simulink library "commdigpbndcpm2"  (Simulink 5.0)
undefined symbols (not defined in the file or in its folder): D
libraries: commblksprivate x14, dspsigattribs x8, commdigbbndcpm2 x8, dspsigops x4, commdigpbndfm2 x2
settings Model: RequirementInfo=9  CovMetricSettings=d  Creator=tdelve  LastModifiedBy=mmclerno

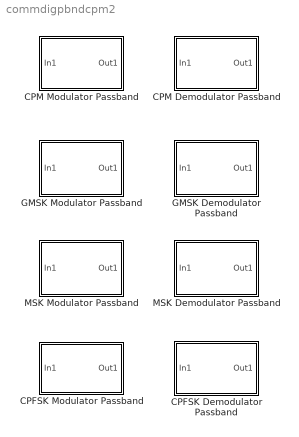
== system commdigpbndcpm2 ==
  CPFSK Demodulator Passband : Subsystem  mask(CPFSK Demodulator Passband){Mnum=4, outputType=Integer, mappingType=Binary, modIdx=.5, td=1/100, numSamp=8, Fc=3000, Ph=0, InSamp=1/8000, traceBack=16}
      mask prompts: Mnum "M-ary number:"; outputType "Output type:"; mappingType "Symbol set ordering:"; modIdx "Modulation index:"; td "Symbol period (s):"; numSamp "Baseband samples per symbol:"; Fc "Carrier frequency (Hz):"; Ph "Carrier initial phase (rad):"; InSamp "Input sample time (s):"; traceBack "Traceback length:"
      mask help:
      | Demodulate the CPFSK modulated input signal using the Viterbi algorithm. Traceback length is the number of trellis branches that the algorithm uses to construct each traceback path.
      |
      | The input must be sample-based.
      |
      | The symbol period divided by the baseband samples per symbol must be an integer multiple of the input sample time.
      mask init:
      | [eStr,params]=commblkpbndcpfskdemod(gcb, 'init');
      | if(eStr.ecode==1)
      |     error(eStr.emsg);
      | elseif(eStr.ecode==2)
      |     warning(eStr.emsg);
      | end;
      settings: RTWFcnNameOpts=Auto  RTWFileNameOpts=Auto
      mask Help: helpview(commbhelp)
      mask StyleString: edit,popup(Bit|Integer),popup(Binary|Gray),edit,edit,edit,edit,edit,edit,edit
      mask CallbackString: |commblkpbndcpfskdemod(gcb,'cbOutputType');||||||||
      mask Display:
      | plot(0,0,100,100,[5+1.5*[[0:.8:10] [10:1.6:20] [20:.8:30]] 50 50 50 50+15*[0 1 1 2 2 3]],[85+10*[sin([0:.8:10]*pi*2/5) sin([10:1.6:20]*pi/5) sin([20:.8:30]*pi*2/5)] 85 99 75 85+8*[1 1 -1 -1 1 1]]);
      | text(50,50,'CPFSK','horiz','center','verti','middle');
  CPFSK Modulator Passband : Subsystem  mask(CPFSK Modulator Passband){Mnum=4, inputType=Integer, mappingType=Binary, modIdx=.5, td=1/100, numSamp=8, Fc=3000, Ph=0, OutSamp=1/8000}
      mask prompts: Mnum "M-ary number:"; inputType "Input type:"; mappingType "Symbol set ordering:"; modIdx "Modulation index:"; td "Symbol period (s):"; numSamp "Baseband samples per symbol:"; Fc "Carrier frequency (Hz):"; Ph "Carrier initial phase (rad):"; OutSamp "Output sample time (s):"
      mask help:
      | Modulate the input signal using continuous phase FSK.
      |
      | The input must be sample-based and contain either an integer or log2(M) bits.
      |
      | The input sample time must equal the symbol period.  Also, the symbol period divided by the baseband samples per symbol must be an integer multiple of the output sample time.
      mask init:
      | [eStr,params]=commblkpbndcpfskmod(gcb, 'init');
      | if(eStr.ecode==1)
      |     error(eStr.emsg);
      | elseif(eStr.ecode==2)
      |     warning(eStr.emsg);
      | end;
      settings: ErrorFcn=commblkpbndcpfskmod  RTWFcnNameOpts=Auto  RTWFileNameOpts=Auto
      mask Help: helpview(commbhelp)
      mask StyleString: edit,popup(Bit|Integer),popup(Binary|Gray),edit,edit,edit,edit,edit,edit
      mask CallbackString: |commblkpbndcpfskmod(gcb,'cbInputType');|||||||
      mask Display:
      | plot(0,0,100,100,[5+15*[0 1 1 2 2 3] 50 50 50 50+1.5*[[0:.8:10] [10:1.6:20] [20:.8:30]]],[85+8*[1 1 -1 -1 1 1] 85 99 75 85+10*[sin([0:.8:10]*pi*2/5) sin([10:1.6:20]*pi/5) sin([20:.8:30]*pi*2/5)]]);
      | text(50,50,'CPFSK','horiz','center','verti','middle');
  CPM Demodulator Passband : Subsystem  mask(CPM Demodulator Passband){Mnum=2, outputType=Integer, mappingType=Binary, modIdx=0.5, pulseShape=Rectangular, BT=0.3, mainLobePulseLength=1, rollOff=0.2, pulseLength=1, preHistory=1, td=1/100, numSamp=8, Fc=3000, Ph=0, InSamp=1/8000, traceBack=16}
      mask prompts: Mnum "M-ary number:"; outputType "Output type:"; mappingType "Symbol set ordering:"; modIdx "Modulation index:"; pulseShape "Frequency pulse shape:"; BT "BT product:"; mainLobePulseLength "Main lobe pulse duration (symbol intervals):"; pulseLength "Pulse length (symbol intervals):"; preHistory "Symbol prehistory:"; td "Symbol period (s):"; numSamp "Baseband samples per symbol:"; Fc "Carrier frequency (Hz):"; Ph "Carrier initial phase (rad):"; InSamp "Input sample time (s):"; traceBack "Traceback length:"
      mask help:
      | Demodulate the CPM modulated input signal using the Viterbi algorithm. Traceback length is the number of trellis branches that the algorithm uses to construct each traceback path.
      |
      | The input must be sample-based.
      |
      | The symbol period divided by the baseband samples per symbol must be an integer multiple of the input sample time.
      mask init:
      | [eStr,params]=commblkpbndcpmdemod(gcb, 'init');
      | if(eStr.ecode==1)
      |     error(eStr.emsg);
      | elseif(eStr.ecode==2)
      |     warning(eStr.emsg);
      | end;
      settings: ErrorFcn=commblkpbndcpmdemod  RTWFcnNameOpts=Auto  RTWFileNameOpts=Auto
      mask Help: helpview(commbhelp)
      mask StyleString: edit,popup(Bit|Integer),popup(Binary|Gray),edit,popup(Rectangular|Raised Cosine|Spectral Raised Cosine|Gaussian|Tamed FM),edit,edit,edit,edit,edit,edit,edit,edit,edit,edit,edit
      mask CallbackString: |commblkpbndcpmdemod(gcb,'cbOutputType');|||commblkpbndcpmdemod(gcb,'cbPulseShape');|||||||||||
      mask Display:
      | plot(0,0,100,100,[5+1.5*[[0:.8:10] [10:1.6:20] [20:.8:30]] 50 50 50 50+15*[0 1 1 2 2 3]],[85+10*[sin([0:.8:10]*pi*2/5) sin([10:1.6:20]*pi/5) sin([20:.8:30]*pi*2/5)] 85 99 75 85+8*[1 1 -1 -1 1 1]]);
      | text(50,50,'CPM','horiz','center','verti','middle');
  CPM Modulator Passband : Subsystem  mask(CPM Modulator Passband){Mnum=2, inputType=Integer, mappingType=Binary, modIdx=0.5, pulseShape=Rectangular, BT=0.3, mainLobePulseLength=1, rollOff=0.2, pulseLength=1, preHistory=1, td=1/100, numSamp=8, Fc=3000, Ph=0, OutSamp=1/8000}
      mask prompts: Mnum "M-ary number:"; inputType "Input type:"; mappingType "Symbol set ordering:"; modIdx "Modulation index:"; pulseShape "Frequency pulse shape:"; BT "BT product:"; mainLobePulseLength "Main lobe pulse duration (symbol intervals):"; pulseLength "Pulse length (symbol intervals):"; preHistory "Symbol prehistory:"; td "Symbol period (s):"; numSamp "Baseband samples per symbol:"; Fc "Carrier frequency (Hz):"; Ph "Carrier initial phase (rad):"; OutSamp "Output sample time (s):"
      mask help:
      | Output the complex envelope representation of the selected continuous phase modulation in response to the input data.
      |
      | The input must be sample-based and contain either an integer or log2(M) bits.
      |
      | The input sample time must equal the symbol period.  Also, the symbol period divided by the baseband samples per symbol must be an integer multiple of the output sample time.
      mask init:
      | [eStr,params]=commblkpbndcpmmod(gcb, 'init');
      | if(eStr.ecode==1)
      |     error(eStr.emsg);
      | elseif(eStr.ecode==2)
      |     warning(eStr.emsg);
      | end;
      settings: ErrorFcn=commblkpbndcpmmod  RTWFcnNameOpts=Auto  RTWFileNameOpts=Auto
      mask Help: helpview(commbhelp)
      mask StyleString: edit,popup(Bit|Integer),popup(Binary|Gray),edit,popup(Rectangular|Raised Cosine|Spectral Raised Cosine|Gaussian|Tamed FM),edit,edit,edit,edit,edit,edit,edit,edit,edit,edit
      mask CallbackString: |commblkpbndcpmmod(gcb,'cbInputType');|||commblkpbndcpmmod(gcb,'cbPulseShape');||||||||||
      mask Display:
      | plot(0,0,100,100,[5+15*[0 1 1 2 2 3] 50 50 50 50+1.5*[[0:.8:10] [10:1.6:20] [20:.8:30]]],[85+8*[1 1 -1 -1 1 1] 85 99 75 85+10*[sin([0:.8:10]*pi*2/5) sin([10:1.6:20]*pi/5) sin([20:.8:30]*pi*2/5)]]);
      | text(50,50,'CPM','horiz','center','verti','middle');
  GMSK Demodulator Passband : Subsystem  mask(GMSK Demodulator Passband){outputType=Integer, BT=.3, pulseLength=4, preHistory=1, td=1/100, numSamp=8, Fc=3000, Ph=0, InSamp=1/8000, traceBack=16}
      mask prompts: outputType "Output type:"; BT "BT product:"; pulseLength "Pulse length (symbol intervals):"; preHistory "Symbol prehistory:"; td "Symbol period (s):"; numSamp "Baseband samples per symbol:"; Fc "Carrier frequency (Hz):"; Ph "Carrier initial phase (rad):"; InSamp "Input sample time (s):"; traceBack "Traceback length:"
      mask help:
      | Demodulate the GMSK modulated input signal using the Viterbi algorithm. Traceback length is the number of trellis branches that the algorithm uses to construct each traceback path.
      |
      | The input must be sample-based.
      |
      | The symbol period divided by the baseband samples per symbol must be an integer multiple of the input sample time.
      mask init:
      | [eStr,params]=commblkpbndgmskdemod(gcb, 'init');
      | if(eStr.ecode==1)
      |     error(eStr.emsg);
      | elseif(eStr.ecode==2)
      |     warning(eStr.emsg);
      | end;
      settings: RTWFcnNameOpts=Auto  RTWFileNameOpts=Auto
      mask Help: helpview(commbhelp)
      mask StyleString: popup(Bit|Integer),edit,edit,edit,edit,edit,edit,edit,edit,edit
      mask Display:
      | plot(0,0,100,100,[5+1.5*[[0:.8:10] [10:1.6:20] [20:.8:30]] 50 50 50 50+15*[0 1 1 2 2 3]],[85+10*[sin([0:.8:10]*pi*2/5) sin([10:1.6:20]*pi/5) sin([20:.8:30]*pi*2/5)] 85 99 75 85+8*[1 1 -1 -1 1 1]]);
      | text(50,50,'GMSK','horiz','center','verti','middle');
  GMSK Modulator Passband : Subsystem  mask(GMSK Modulator Passband){inputType=Integer, BT=.3, pulseLength=4, preHistory=1, td=1/100, numSamp=8, Fc=3000, Ph=0, OutSamp=1/8000}
      mask prompts: inputType "Input type:"; BT "BT product:"; pulseLength "Pulse length (symbol intervals):"; preHistory "Symbol prehistory:"; td "Symbol period (s):"; numSamp "Baseband samples per symbol:"; Fc "Carrier frequency (Hz):"; Ph "Carrier initial phase (rad):"; OutSamp "Output sample time (s):"
      mask help:
      | Modulate the input signal using GMSK.
      |
      | The input must be sample-based and contain either an integer or log2(M) bits.
      |
      | The input sample time must equal the symbol period.  Also, the symbol period divided by the baseband samples per symbol must be an integer multiple of the output sample time.
      mask init:
      | [eStr,params]=commblkpbndgmskmod(gcb, 'init');
      | if(eStr.ecode==1)
      |     error(eStr.emsg);
      | elseif(eStr.ecode==2)
      |     warning(eStr.emsg);
      | end;
      settings: ErrorFcn=commblkpbndgmskmod  RTWFcnNameOpts=Auto  RTWFileNameOpts=Auto
      mask Help: helpview(commbhelp)
      mask StyleString: popup(Bit|Integer),edit,edit,edit,edit,edit,edit,edit,edit
      mask Display:
      | plot(0,0,100,100,[5+15*[0 1 1 2 2 3] 50 50 50 50+1.5*[[0:.8:10] [10:1.6:20] [20:.8:30]]],[85+8*[1 1 -1 -1 1 1] 85 99 75 85+10*[sin([0:.8:10]*pi*2/5) sin([10:1.6:20]*pi/5) sin([20:.8:30]*pi*2/5)]]);
      | text(50,50,'GMSK','horiz','center','verti','middle');
  MSK Demodulator Passband : Subsystem  mask(MSK Demodulator Passband){outputType=Integer, td=1/100, numSamp=8, Fc=3000, Ph=0, InSamp=1/8000, traceBack=16}
      mask prompts: outputType "Output type:"; td "Symbol period (s):"; numSamp "Baseband samples per symbol:"; Fc "Carrier frequency (Hz):"; Ph "Carrier initial phase (rad):"; InSamp "Input sample time (s):"; traceBack "Traceback length:"
      mask help:
      | Demodulate the MSK modulated input signal using the Viterbi algorithm. Traceback length is the number of trellis branches that the algorithm uses to construct each traceback path.
      |
      | The input must be sample-based.
      |
      | The symbol period divided by the baseband samples per symbol must be an integer multiple of the input sample time.
      mask init:
      | [eStr,params]=commblkpbndmskdemod(gcb, 'init');
      | if(eStr.ecode==1)
      |     error(eStr.emsg);
      | elseif(eStr.ecode==2)
      |     warning(eStr.emsg);
      | end;
      settings: RTWFcnNameOpts=Auto  RTWFileNameOpts=Auto
      mask Help: helpview(commbhelp)
      mask StyleString: popup(Bit|Integer),edit,edit,edit,edit,edit,edit
      mask Display:
      | plot(0,0,100,100,[5+1.5*[[0:.8:10] [10:1.6:20] [20:.8:30]] 50 50 50 50+15*[0 1 1 2 2 3]],[85+10*[sin([0:.8:10]*pi*2/5) sin([10:1.6:20]*pi/5) sin([20:.8:30]*pi*2/5)] 85 99 75 85+8*[1 1 -1 -1 1 1]]);
      | text(51,51,'MSK','horiz','center','verti','middle');
  MSK Modulator Passband : Subsystem  mask(MSK Modulator Passband){inputType=Integer, td=1/100, numSamp=8, Fc=3000, Ph=0, OutSamp=1/8000}
      mask prompts: inputType "Input type:"; td "Symbol period (s):"; numSamp "Baseband samples per symbol:"; Fc "Carrier frequency (Hz):"; Ph "Carrier initial phase (rad):"; OutSamp "Output sample time (s):"
      mask help:
      | Modulate the input signal using MSK.
      |
      | The input must be sample-based and contain either an integer or log2(M) bits.
      |
      | The input sample time must equal the symbol period.  Also, the symbol period divided by the baseband samples per symbol must be an integer multiple of the output sample time.
      mask init:
      | [eStr,params]=commblkpbndmskmod(gcb, 'init');
      | if(eStr.ecode==1)
      |     error(eStr.emsg);
      | elseif(eStr.ecode==2)
      |     warning(eStr.emsg);
      | end;
      settings: ErrorFcn=commblkpbndmskmod  RTWFcnNameOpts=Auto  RTWFileNameOpts=Auto
      mask Help: helpview(commbhelp)
      mask StyleString: popup(Bit|Integer),edit,edit,edit,edit,edit
      mask Display:
      | plot(0,0,100,100,[5+15*[0 1 1 2 2 3] 50 50 50 50+1.5*[[0:.8:10] [10:1.6:20] [20:.8:30]]],[85+8*[1 1 -1 -1 1 1] 85 99 75 85+10*[sin([0:.8:10]*pi*2/5) sin([10:1.6:20]*pi/5) sin([20:.8:30]*pi*2/5)]]);
      | text(51,51,'MSK','horiz','center','verti','middle');

== system commdigpbndcpm2/CPFSK Demodulator Passband ==
  In1 : Inport  Port=1  LatchInput=off
  CPM Demodulator Passband : Subsystem  AncestorBlock=|  mask(CPM Demodulator Passband){Mnum=Mnum, outputType=Integer, mappingType=Binary, modIdx=modIdx, pulseShape=Rectangular, BT=0.3, mainLobePulseLength=1, rollOff=0.2, pulseLength=1, preHistory=1, td=td, numSamp=numSamp, Fc=Fc, Ph=Ph, InSamp=InSamp, traceBack=traceBack}
      | commdigpbndcpm2/CPM
      | Demodulator
      | Passband
      mask prompts: Mnum "M-ary number:"; outputType "Output type:"; mappingType "Symbol set ordering:"; modIdx "Modulation index:"; pulseShape "Frequency pulse shape:"; BT "BT product:"; mainLobePulseLength "Main lobe pulse duration (symbol intervals):"; pulseLength "Pulse length (symbol intervals):"; preHistory "Symbol prehistory:"; td "Symbol period (s):"; numSamp "Baseband samples per symbol:"; Fc "Carrier frequency (Hz):"; Ph "Carrier initial phase (rad):"; InSamp "Input sample time (s):"; traceBack "Traceback length:"
      mask help:
      | Demodulate the CPM modulated input signal using the Viterbi algorithm. Traceback length is the number of trellis branches that the algorithm uses to construct each traceback path.
      |
      | The input must be sample-based.
      mask init:
      | [eStr,params]=commblkpbndcpmdemod(gcb, 'init');
      | if(eStr.ecode==1)
      |     error(eStr.emsg);
      | elseif(eStr.ecode==2)
      |     warning(eStr.emsg);
      | end;
      settings: ErrorFcn=commblkpbndcpmdemod  RTWFcnNameOpts=Auto  RTWFileNameOpts=Auto
      mask Help: helpview(commbhelp)
      mask StyleString: edit,popup(Bit|Integer),popup(Binary|Gray),edit,popup(Rectangular|Raised Cosine|Spectral Raised Cosine|Gaussian|Tamed FM),edit,edit,edit,edit,edit,edit,edit,edit,edit,edit,edit
      mask CallbackString: |commblkpbndcpmdemod(gcb,'cbOutputType');|||commblkpbndcpmdemod(gcb,'cbPulseShape');|||||||||||
      mask Display:
      | plot(0,0,100,100,[5+1.5*[[0:.8:10] [10:1.6:20] [20:.8:30]] 50 50 50 50+15*[0 1 1 2 2 3]],[85+10*[sin([0:.8:10]*pi*2/5) sin([10:1.6:20]*pi/5) sin([20:.8:30]*pi*2/5)] 85 99 75 85+8*[1 1 -1 -1 1 1]]);
      | text(50,50,'CPM','horiz','center','verti','middle');
  Out1 : Outport  Port=1
  wires:
  CPM Demodulator Passband/1(Out1) -> Out1/1
  In1/1 -> CPM Demodulator Passband/1(In1)

== system commdigpbndcpm2/CPFSK Modulator Passband ==
  In1 : Inport  Port=1  LatchInput=off
  CPM Modulator Passband : Subsystem  AncestorBlock=|  mask(CPM Modulator Passband){Mnum=Mnum, inputType=Integer, mappingType=Binary, modIdx=modIdx, pulseShape=Rectangular, BT=0.3, mainLobePulseLength=1, rollOff=0.2, pulseLength=1, preHistory=1, td=td, numSamp=numSamp, Fc=Fc, Ph=Ph, OutSamp=OutSamp}
      | commdigpbndcpm2/CPM
      | Modulator
      | Passband
      mask prompts: Mnum "M-ary number:"; inputType "Input type:"; mappingType "Symbol set ordering:"; modIdx "Modulation index:"; pulseShape "Frequency pulse shape:"; BT "BT product:"; mainLobePulseLength "Main lobe pulse duration (symbol intervals):"; pulseLength "Pulse length (symbol intervals):"; preHistory "Symbol prehistory:"; td "Symbol period (s):"; numSamp "Baseband samples per symbol:"; Fc "Carrier frequency (Hz):"; Ph "Carrier initial phase (rad):"; OutSamp "Output sample time:"
      mask help:
      | Output the complex envelope representation of the selected continuous phase modulation in response to the input data.
      |
      | The input must be sample-based and contain either an integer or log2(M) bits. The input sample time must equal the symbol period.
      mask init:
      | [eStr,params]=commblkpbndcpmmod(gcb, 'init');
      | if(eStr.ecode==1)
      |     error(eStr.emsg);
      | elseif(eStr.ecode==2)
      |     warning(eStr.emsg);
      | end;
      settings: ErrorFcn=commblkpbndcpmmod  RTWFcnNameOpts=Auto  RTWFileNameOpts=Auto
      mask Help: helpview(commbhelp)
      mask StyleString: edit,popup(Bit|Integer),popup(Binary|Gray),edit,popup(Rectangular|Raised Cosine|Spectral Raised Cosine|Gaussian|Tamed FM),edit,edit,edit,edit,edit,edit,edit,edit,edit,edit
      mask CallbackString: |commblkpbndcpmmod(gcb,'cbInputType');|||commblkpbndcpmmod(gcb,'cbPulseShape');||||||||||
      mask Display:
      | plot(0,0,100,100,[5+15*[0 1 1 2 2 3] 50 50 50 50+1.5*[[0:.8:10] [10:1.6:20] [20:.8:30]]],[85+8*[1 1 -1 -1 1 1] 85 99 75 85+10*[sin([0:.8:10]*pi*2/5) sin([10:1.6:20]*pi/5) sin([20:.8:30]*pi*2/5)]]);
      | text(50,50,'CPM','horiz','center','verti','middle');
  Out1 : Outport  Port=1
  wires:
  CPM Modulator Passband/1(Out1) -> Out1/1
  In1/1 -> CPM Modulator Passband/1(In1)

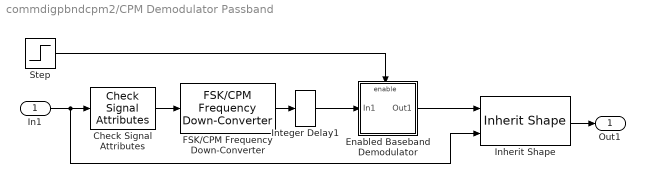
== system commdigpbndcpm2/CPM Demodulator Passband ==
  In1 : Inport  Port=1  LatchInput=off
  Check Signal Attributes : dspsigattribs/Check Signal Attributes  SigAttribCheckMethod=Matches attributes exactly  Complexity=Ignore  Frame=Frame-based  DimsCheckMethod=Ignore  Dimensions=1-D  DatatypeCheckMethod=Ignore  DatatypeGeneral=Boolean  DtypeFloatSpecific=Any floating-point  DtypeFixedSpecific=Any fixed-point  DtypeIntSpecific=Any integer  SampleMode=Ignore
  Enabled Baseband Demodulator : Subsystem  TreatAsAtomicUnit=on
      settings: RTWFcnNameOpts=Auto  RTWFileNameOpts=Auto
  FSK/CPM Frequency Down-Converter : commblksprivate/FSK//CPM Frequency Down-Converter  modType=CPM  M=8  freqSep=100  td=td  Fc=Fc  Ph=Ph  Tin=InSamp  Tout=td / numSamp
  Inherit Shape : commblksprivate/Inherit Shape
  Integer Delay1 : dspsigops/Integer Delay  delay=numSamp-1  ic=0
  Step : Step  Time=td  Before=0  After=1  SampleTime=td
  Out1 : Outport  Port=1
  wires:
  Check Signal Attributes/1 -> FSK/CPM Frequency Down-Converter/1
  FSK/CPM Frequency Down-Converter/1 -> Integer Delay1/1
  Enabled Baseband Demodulator/1(Out1) -> Inherit Shape/1
  In1/1 -> Check Signal Attributes/1, Inherit Shape/2
  Inherit Shape/1 -> Out1/1
  Integer Delay1/1 -> Enabled Baseband Demodulator/1(In1)
  Step/1 -> Enabled Baseband Demodulator/Enable

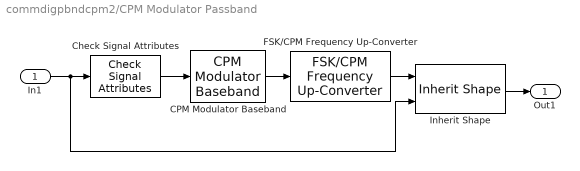
== system commdigpbndcpm2/CPM Modulator Passband ==
  In1 : Inport  Port=1  LatchInput=off
  CPM Modulator Baseband : commdigbbndcpm2/CPM Modulator Baseband  Mnum=Mnum  inputType=Integer  mappingType=Binary  modIdx=modIdx  pulseShape=Rectangular  BT=BT  mainLobePulseLength=1  rollOff=rollOff  pulseLength=pulseLength  preHistory=preHistory  phaseOffset=0  samplesPerSymbol=numSamp
  Check Signal Attributes : dspsigattribs/Check Signal Attributes  SigAttribCheckMethod=Matches attributes exactly  Complexity=Ignore  Frame=Frame-based  DimsCheckMethod=Ignore  Dimensions=1-D  DatatypeCheckMethod=Ignore  DatatypeGeneral=Boolean  DtypeFloatSpecific=Any floating-point  DtypeFixedSpecific=Any fixed-point  DtypeIntSpecific=Any integer  SampleMode=Ignore
  FSK/CPM Frequency Up-Converter : commblksprivate/FSK//CPM Frequency Up-Converter  modType=CPM  M=8  freqSep=6  td=td  Fc=Fc  Ph=Ph  Tin=td / numSamp  Tout=OutSamp
  Inherit Shape : commblksprivate/Inherit Shape
  Out1 : Outport  Port=1
  wires:
  FSK/CPM Frequency Up-Converter/1 -> Inherit Shape/1
  CPM Modulator Baseband/1 -> FSK/CPM Frequency Up-Converter/1
  Check Signal Attributes/1 -> CPM Modulator Baseband/1
  In1/1 -> Check Signal Attributes/1, Inherit Shape/2
  Inherit Shape/1 -> Out1/1

== system commdigpbndcpm2/GMSK Demodulator Passband ==
  In1 : Inport  Port=1  LatchInput=off
  CPM Demodulator Passband : Subsystem  AncestorBlock=|  mask(CPM Demodulator Passband){Mnum=2, outputType=Integer, mappingType=Binary, modIdx=0.5, pulseShape=Gaussian, BT=BT, mainLobePulseLength=1, rollOff=0.2, pulseLength=pulseLength, preHistory=preHistory, td=td, numSamp=numSamp, Fc=Fc, Ph=Ph, InSamp=InSamp, traceBack=traceBack}
      | commdigpbndcpm2/CPM
      | Demodulator
      | Passband
      mask prompts: Mnum "M-ary number:"; outputType "Output type:"; mappingType "Symbol set ordering:"; modIdx "Modulation index:"; pulseShape "Frequency pulse shape:"; BT "BT product:"; mainLobePulseLength "Main lobe pulse duration (symbol intervals):"; pulseLength "Pulse length (symbol intervals):"; preHistory "Symbol prehistory:"; td "Symbol period (s):"; numSamp "Baseband samples per symbol:"; Fc "Carrier frequency (Hz):"; Ph "Carrier initial phase (rad):"; InSamp "Input sample time (s):"; traceBack "Traceback length:"
      mask help:
      | Demodulate the CPM modulated input signal using the Viterbi algorithm. Traceback length is the number of trellis branches that the algorithm uses to construct each traceback path.
      |
      | The input must be sample-based.
      mask init:
      | [eStr,params]=commblkpbndcpmdemod(gcb, 'init');
      | if(eStr.ecode==1)
      |     error(eStr.emsg);
      | elseif(eStr.ecode==2)
      |     warning(eStr.emsg);
      | end;
      settings: ErrorFcn=commblkpbndcpmdemod  RTWFcnNameOpts=Auto  RTWFileNameOpts=Auto
      mask Help: helpview(commbhelp)
      mask StyleString: edit,popup(Bit|Integer),popup(Binary|Gray),edit,popup(Rectangular|Raised Cosine|Spectral Raised Cosine|Gaussian|Tamed FM),edit,edit,edit,edit,edit,edit,edit,edit,edit,edit,edit
      mask CallbackString: |commblkpbndcpmdemod(gcb,'cbOutputType');|||commblkpbndcpmdemod(gcb,'cbPulseShape');|||||||||||
      mask Display:
      | plot(0,0,100,100,[5+1.5*[[0:.8:10] [10:1.6:20] [20:.8:30]] 50 50 50 50+15*[0 1 1 2 2 3]],[85+10*[sin([0:.8:10]*pi*2/5) sin([10:1.6:20]*pi/5) sin([20:.8:30]*pi*2/5)] 85 99 75 85+8*[1 1 -1 -1 1 1]]);
      | text(50,50,'CPM','horiz','center','verti','middle');
  Out1 : Outport  Port=1
  wires:
  CPM Demodulator Passband/1(Out1) -> Out1/1
  In1/1 -> CPM Demodulator Passband/1(In1)

== system commdigpbndcpm2/GMSK Modulator Passband ==
  In1 : Inport  Port=1  LatchInput=off
  CPM Modulator Passband : Subsystem  AncestorBlock=|  mask(CPM Modulator Passband){Mnum=2, inputType=Integer, mappingType=Binary, modIdx=.5, pulseShape=Gaussian, BT=BT, mainLobePulseLength=1, rollOff=0.2, pulseLength=pulseLength, preHistory=preHistory, td=td, numSamp=numSamp, Fc=Fc, Ph=Ph, OutSamp=OutSamp}
      | commdigpbndcpm2/CPM
      | Modulator
      | Passband
      mask prompts: Mnum "M-ary number:"; inputType "Input type:"; mappingType "Symbol set ordering:"; modIdx "Modulation index:"; pulseShape "Frequency pulse shape:"; BT "BT product:"; mainLobePulseLength "Main lobe pulse duration (symbol intervals):"; pulseLength "Pulse length (symbol intervals):"; preHistory "Symbol prehistory:"; td "Symbol period (s):"; numSamp "Baseband samples per symbol:"; Fc "Carrier frequency (Hz):"; Ph "Carrier initial phase (rad):"; OutSamp "Output sample time:"
      mask help:
      | Output the complex envelope representation of the selected continuous phase modulation in response to the input data.
      |
      | The input must be sample-based and contain either an integer or log2(M) bits. The input sample time must equal the symbol period.
      mask init:
      | [eStr,params]=commblkpbndcpmmod(gcb, 'init');
      | if(eStr.ecode==1)
      |     error(eStr.emsg);
      | elseif(eStr.ecode==2)
      |     warning(eStr.emsg);
      | end;
      settings: ErrorFcn=commblkpbndcpmmod  RTWFcnNameOpts=Auto  RTWFileNameOpts=Auto
      mask Help: helpview(commbhelp)
      mask StyleString: edit,popup(Bit|Integer),popup(Binary|Gray),edit,popup(Rectangular|Raised Cosine|Spectral Raised Cosine|Gaussian|Tamed FM),edit,edit,edit,edit,edit,edit,edit,edit,edit,edit
      mask CallbackString: |commblkpbndcpmmod(gcb,'cbInputType');|||commblkpbndcpmmod(gcb,'cbPulseShape');||||||||||
      mask Display:
      | plot(0,0,100,100,[5+15*[0 1 1 2 2 3] 50 50 50 50+1.5*[[0:.8:10] [10:1.6:20] [20:.8:30]]],[85+8*[1 1 -1 -1 1 1] 85 99 75 85+10*[sin([0:.8:10]*pi*2/5) sin([10:1.6:20]*pi/5) sin([20:.8:30]*pi*2/5)]]);
      | text(50,50,'CPM','horiz','center','verti','middle');
  Out1 : Outport  Port=1
  wires:
  CPM Modulator Passband/1(Out1) -> Out1/1
  In1/1 -> CPM Modulator Passband/1(In1)

== system commdigpbndcpm2/MSK Demodulator Passband ==
  In1 : Inport  Port=1  LatchInput=off
  CPM Demodulator Passband : Subsystem  AncestorBlock=|  mask(CPM Demodulator Passband){Mnum=2, outputType=Integer, mappingType=Binary, modIdx=0.5, pulseShape=Rectangular, BT=0.3, mainLobePulseLength=1, rollOff=0.2, pulseLength=1, preHistory=1, td=td, numSamp=numSamp, Fc=Fc, Ph=Ph, InSamp=InSamp, traceBack=traceBack}
      | commdigpbndcpm2/CPM
      | Demodulator
      | Passband
      mask prompts: Mnum "M-ary number:"; outputType "Output type:"; mappingType "Symbol set ordering:"; modIdx "Modulation index:"; pulseShape "Frequency pulse shape:"; BT "BT product:"; mainLobePulseLength "Main lobe pulse duration (symbol intervals):"; pulseLength "Pulse length (symbol intervals):"; preHistory "Symbol prehistory:"; td "Symbol period (s):"; numSamp "Baseband samples per symbol:"; Fc "Carrier frequency (Hz):"; Ph "Carrier initial phase (rad):"; InSamp "Input sample time (s):"; traceBack "Traceback length:"
      mask help:
      | Demodulate the CPM modulated input signal using the Viterbi algorithm. Traceback length is the number of trellis branches that the algorithm uses to construct each traceback path.
      |
      | The input must be sample-based.
      mask init:
      | [eStr,params]=commblkpbndcpmdemod(gcb, 'init');
      | if(eStr.ecode==1)
      |     error(eStr.emsg);
      | elseif(eStr.ecode==2)
      |     warning(eStr.emsg);
      | end;
      settings: ErrorFcn=commblkpbndcpmdemod  RTWFcnNameOpts=Auto  RTWFileNameOpts=Auto
      mask Help: helpview(commbhelp)
      mask StyleString: edit,popup(Bit|Integer),popup(Binary|Gray),edit,popup(Rectangular|Raised Cosine|Spectral Raised Cosine|Gaussian|Tamed FM),edit,edit,edit,edit,edit,edit,edit,edit,edit,edit,edit
      mask CallbackString: |commblkpbndcpmdemod(gcb,'cbOutputType');|||commblkpbndcpmdemod(gcb,'cbPulseShape');|||||||||||
      mask Display:
      | plot(0,0,100,100,[5+1.5*[[0:.8:10] [10:1.6:20] [20:.8:30]] 50 50 50 50+15*[0 1 1 2 2 3]],[85+10*[sin([0:.8:10]*pi*2/5) sin([10:1.6:20]*pi/5) sin([20:.8:30]*pi*2/5)] 85 99 75 85+8*[1 1 -1 -1 1 1]]);
      | text(50,50,'CPM','horiz','center','verti','middle');
  Out1 : Outport  Port=1
  wires:
  CPM Demodulator Passband/1(Out1) -> Out1/1
  In1/1 -> CPM Demodulator Passband/1(In1)

== system commdigpbndcpm2/MSK Modulator Passband ==
  In1 : Inport  Port=1  LatchInput=off
  CPM Modulator Passband : Subsystem  AncestorBlock=|  mask(CPM Modulator Passband){Mnum=2, inputType=Integer, mappingType=Binary, modIdx=0.5, pulseShape=Rectangular, BT=0.3, mainLobePulseLength=1, rollOff=0.2, pulseLength=1, preHistory=1, td=td, numSamp=numSamp, Fc=Fc, Ph=Ph, OutSamp=OutSamp}
      | commdigpbndcpm2/CPM
      | Modulator
      | Passband
      mask prompts: Mnum "M-ary number:"; inputType "Input type:"; mappingType "Symbol set ordering:"; modIdx "Modulation index:"; pulseShape "Frequency pulse shape:"; BT "BT product:"; mainLobePulseLength "Main lobe pulse duration (symbol intervals):"; pulseLength "Pulse length (symbol intervals):"; preHistory "Symbol prehistory:"; td "Symbol period (s):"; numSamp "Baseband samples per symbol:"; Fc "Carrier frequency (Hz):"; Ph "Carrier initial phase (rad):"; OutSamp "Output sample time:"
      mask help:
      | Output the complex envelope representation of the selected continuous phase modulation in response to the input data.
      |
      | The input must be sample-based and contain either an integer or log2(M) bits. The input sample time must equal the symbol period.
      mask init:
      | [eStr,params]=commblkpbndcpmmod(gcb, 'init');
      | if(eStr.ecode==1)
      |     error(eStr.emsg);
      | elseif(eStr.ecode==2)
      |     warning(eStr.emsg);
      | end;
      settings: ErrorFcn=commblkpbndcpmmod  RTWFcnNameOpts=Auto  RTWFileNameOpts=Auto
      mask Help: helpview(commbhelp)
      mask StyleString: edit,popup(Bit|Integer),popup(Binary|Gray),edit,popup(Rectangular|Raised Cosine|Spectral Raised Cosine|Gaussian|Tamed FM),edit,edit,edit,edit,edit,edit,edit,edit,edit,edit
      mask CallbackString: |commblkpbndcpmmod(gcb,'cbInputType');|||commblkpbndcpmmod(gcb,'cbPulseShape');||||||||||
      mask Display:
      | plot(0,0,100,100,[5+15*[0 1 1 2 2 3] 50 50 50 50+1.5*[[0:.8:10] [10:1.6:20] [20:.8:30]]],[85+8*[1 1 -1 -1 1 1] 85 99 75 85+10*[sin([0:.8:10]*pi*2/5) sin([10:1.6:20]*pi/5) sin([20:.8:30]*pi*2/5)]]);
      | text(50,50,'CPM','horiz','center','verti','middle');
  Out1 : Outport  Port=1
  wires:
  CPM Modulator Passband/1(Out1) -> Out1/1
  In1/1 -> CPM Modulator Passband/1(In1)

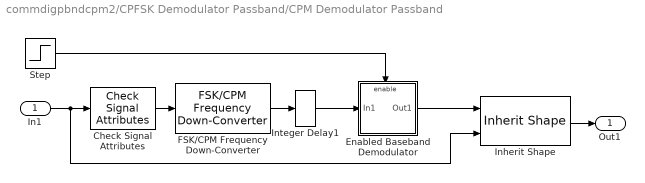
== system commdigpbndcpm2/CPFSK Demodulator Passband/CPM Demodulator Passband ==
  In1 : Inport  Port=1  LatchInput=off
  Check Signal Attributes : dspsigattribs/Check Signal Attributes  SigAttribCheckMethod=Matches attributes exactly  Complexity=Ignore  Frame=Frame-based  DimsCheckMethod=Ignore  Dimensions=1-D  DatatypeCheckMethod=Ignore  DatatypeGeneral=Boolean  DtypeFloatSpecific=Any floating-point  DtypeFixedSpecific=Any fixed-point  DtypeIntSpecific=Any integer  SampleMode=Ignore
  Enabled Baseband Demodulator : Subsystem  TreatAsAtomicUnit=on
      settings: RTWFcnNameOpts=Auto  RTWFileNameOpts=Auto
  FSK/CPM Frequency Down-Converter : commblksprivate/FSK//CPM Frequency Down-Converter  AncestorBlock=|  modType=CPM  M=8  freqSep=100  td=td  Fc=Fc  Ph=Ph  Tin=InSamp  Tout=td / numSamp
      | commblksprivate/PAM//QAM//PSK
      | Frequency
      | Down-Converter
  Inherit Shape : commblksprivate/Inherit Shape
  Integer Delay1 : dspsigops/Integer Delay  delay=numSamp-1  ic=0
  Step : Step  Time=td  Before=0  After=1  SampleTime=td
  Out1 : Outport  Port=1
  wires:
  Step/1 -> Enabled Baseband Demodulator/Enable
  Integer Delay1/1 -> Enabled Baseband Demodulator/1(In1)
  Inherit Shape/1 -> Out1/1
  In1/1 -> Inherit Shape/2, Check Signal Attributes/1
  Enabled Baseband Demodulator/1(Out1) -> Inherit Shape/1
  FSK/CPM Frequency Down-Converter/1 -> Integer Delay1/1
  Check Signal Attributes/1 -> FSK/CPM Frequency Down-Converter/1

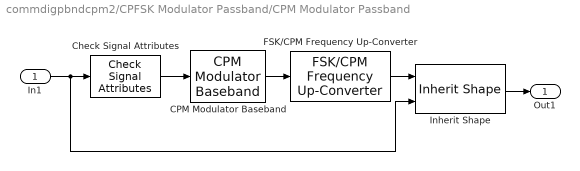
== system commdigpbndcpm2/CPFSK Modulator Passband/CPM Modulator Passband ==
  In1 : Inport  Port=1  LatchInput=off
  CPM Modulator Baseband : commdigbbndcpm2/CPM Modulator Baseband  Mnum=Mnum  inputType=Integer  mappingType=Binary  modIdx=modIdx  pulseShape=Rectangular  BT=BT  mainLobePulseLength=1  rollOff=rollOff  pulseLength=pulseLength  preHistory=preHistory  phaseOffset=0  samplesPerSymbol=numSamp
  Check Signal Attributes : dspsigattribs/Check Signal Attributes  SigAttribCheckMethod=Matches attributes exactly  Complexity=Ignore  Frame=Frame-based  DimsCheckMethod=Ignore  Dimensions=1-D  DatatypeCheckMethod=Ignore  DatatypeGeneral=Boolean  DtypeFloatSpecific=Any floating-point  DtypeFixedSpecific=Any fixed-point  DtypeIntSpecific=Any integer  SampleMode=Ignore
  FSK/CPM Frequency Up-Converter : commdigpbndfm2/M-FSK Modulator Passband/FSK//CPM Frequency Up-Converter  AncestorBlock=|  modType=CPM  M=8  freqSep=6  td=td  Fc=Fc  Ph=Ph  Tin=td / numSamp  Tout=OutSamp
      | commblksprivate/FSK//CPM
      | Frequency
      | Up-Converter
  Inherit Shape : commblksprivate/Inherit Shape
  Out1 : Outport  Port=1
  wires:
  Inherit Shape/1 -> Out1/1
  In1/1 -> Inherit Shape/2, Check Signal Attributes/1
  Check Signal Attributes/1 -> CPM Modulator Baseband/1
  CPM Modulator Baseband/1 -> FSK/CPM Frequency Up-Converter/1
  FSK/CPM Frequency Up-Converter/1 -> Inherit Shape/1

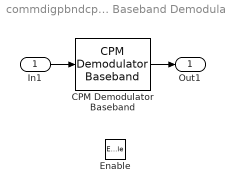
== system commdigpbndcpm2/CPM Demodulator Passband/Enabled Baseband Demodulator ==
  In1 : Inport  Port=1  LatchInput=off
  Enable : EnablePort
  CPM Demodulator Baseband : commdigbbndcpm2/CPM Demodulator Baseband  Mnum=Mnum  outputType=Integer  mappingType=Binary  modIdx=modIdx  pulseShape=Rectangular  BT=BT  mainLobePulseLength=1  rollOff=rollOff  pulseLength=pulseLength  preHistory=preHistory  phaseOffset=0  samplesPerSymbol=numSamp  traceBack=traceBack
  Out1 : Outport  Port=1
  wires:
  CPM Demodulator Baseband/1 -> Out1/1
  In1/1 -> CPM Demodulator Baseband/1

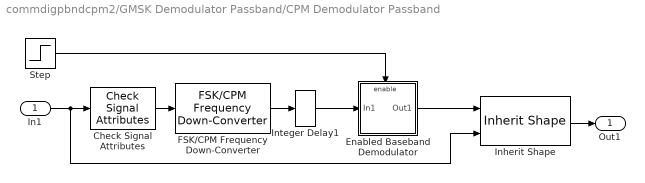
== system commdigpbndcpm2/GMSK Demodulator Passband/CPM Demodulator Passband ==
  In1 : Inport  Port=1  LatchInput=off
  Check Signal Attributes : dspsigattribs/Check Signal Attributes  SigAttribCheckMethod=Matches attributes exactly  Complexity=Ignore  Frame=Frame-based  DimsCheckMethod=Ignore  Dimensions=1-D  DatatypeCheckMethod=Ignore  DatatypeGeneral=Boolean  DtypeFloatSpecific=Any floating-point  DtypeFixedSpecific=Any fixed-point  DtypeIntSpecific=Any integer  SampleMode=Ignore
  Enabled Baseband Demodulator : Subsystem  TreatAsAtomicUnit=on
      settings: RTWFcnNameOpts=Auto  RTWFileNameOpts=Auto
  FSK/CPM Frequency Down-Converter : commblksprivate/FSK//CPM Frequency Down-Converter  AncestorBlock=|  modType=CPM  M=8  freqSep=100  td=td  Fc=Fc  Ph=Ph  Tin=InSamp  Tout=td / numSamp
      | commblksprivate/PAM//QAM//PSK
      | Frequency
      | Down-Converter
  Inherit Shape : commblksprivate/Inherit Shape
  Integer Delay1 : dspsigops/Integer Delay  delay=numSamp-1  ic=0
  Step : Step  Time=td  Before=0  After=1  SampleTime=td
  Out1 : Outport  Port=1
  wires:
  Step/1 -> Enabled Baseband Demodulator/Enable
  Integer Delay1/1 -> Enabled Baseband Demodulator/1(In1)
  Inherit Shape/1 -> Out1/1
  In1/1 -> Inherit Shape/2, Check Signal Attributes/1
  Enabled Baseband Demodulator/1(Out1) -> Inherit Shape/1
  FSK/CPM Frequency Down-Converter/1 -> Integer Delay1/1
  Check Signal Attributes/1 -> FSK/CPM Frequency Down-Converter/1

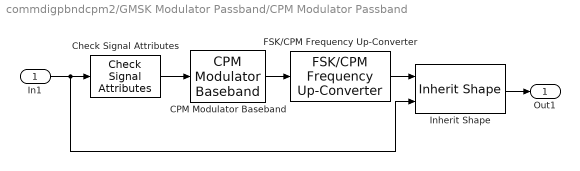
== system commdigpbndcpm2/GMSK Modulator Passband/CPM Modulator Passband ==
  In1 : Inport  Port=1  LatchInput=off
  CPM Modulator Baseband : commdigbbndcpm2/CPM Modulator Baseband  Mnum=Mnum  inputType=Integer  mappingType=Binary  modIdx=modIdx  pulseShape=Gaussian  BT=BT  mainLobePulseLength=1  rollOff=rollOff  pulseLength=pulseLength  preHistory=preHistory  phaseOffset=0  samplesPerSymbol=numSamp
  Check Signal Attributes : dspsigattribs/Check Signal Attributes  SigAttribCheckMethod=Matches attributes exactly  Complexity=Ignore  Frame=Frame-based  DimsCheckMethod=Ignore  Dimensions=1-D  DatatypeCheckMethod=Ignore  DatatypeGeneral=Boolean  DtypeFloatSpecific=Any floating-point  DtypeFixedSpecific=Any fixed-point  DtypeIntSpecific=Any integer  SampleMode=Ignore
  FSK/CPM Frequency Up-Converter : commdigpbndfm2/M-FSK Modulator Passband/FSK//CPM Frequency Up-Converter  AncestorBlock=|  modType=CPM  M=8  freqSep=6  td=td  Fc=Fc  Ph=Ph  Tin=td / numSamp  Tout=OutSamp
      | commblksprivate/FSK//CPM
      | Frequency
      | Up-Converter
  Inherit Shape : commblksprivate/Inherit Shape
  Out1 : Outport  Port=1
  wires:
  Inherit Shape/1 -> Out1/1
  In1/1 -> Inherit Shape/2, Check Signal Attributes/1
  Check Signal Attributes/1 -> CPM Modulator Baseband/1
  CPM Modulator Baseband/1 -> FSK/CPM Frequency Up-Converter/1
  FSK/CPM Frequency Up-Converter/1 -> Inherit Shape/1

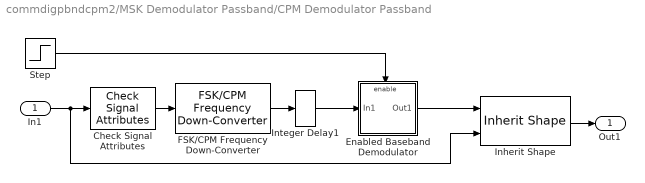
== system commdigpbndcpm2/MSK Demodulator Passband/CPM Demodulator Passband ==
  In1 : Inport  Port=1  LatchInput=off
  Check Signal Attributes : dspsigattribs/Check Signal Attributes  SigAttribCheckMethod=Matches attributes exactly  Complexity=Ignore  Frame=Frame-based  DimsCheckMethod=Ignore  Dimensions=1-D  DatatypeCheckMethod=Ignore  DatatypeGeneral=Boolean  DtypeFloatSpecific=Any floating-point  DtypeFixedSpecific=Any fixed-point  DtypeIntSpecific=Any integer  SampleMode=Ignore
  Enabled Baseband Demodulator : Subsystem  TreatAsAtomicUnit=on
      settings: RTWFcnNameOpts=Auto  RTWFileNameOpts=Auto
  FSK/CPM Frequency Down-Converter : commblksprivate/FSK//CPM Frequency Down-Converter  AncestorBlock=|  modType=CPM  M=8  freqSep=100  td=td  Fc=Fc  Ph=Ph  Tin=InSamp  Tout=td / numSamp
      | commblksprivate/PAM//QAM//PSK
      | Frequency
      | Down-Converter
  Inherit Shape : commblksprivate/Inherit Shape
  Integer Delay1 : dspsigops/Integer Delay  delay=numSamp-1  ic=0
  Step : Step  Time=td  Before=0  After=1  SampleTime=td
  Out1 : Outport  Port=1
  wires:
  Step/1 -> Enabled Baseband Demodulator/Enable
  Integer Delay1/1 -> Enabled Baseband Demodulator/1(In1)
  Inherit Shape/1 -> Out1/1
  In1/1 -> Inherit Shape/2, Check Signal Attributes/1
  Enabled Baseband Demodulator/1(Out1) -> Inherit Shape/1
  FSK/CPM Frequency Down-Converter/1 -> Integer Delay1/1
  Check Signal Attributes/1 -> FSK/CPM Frequency Down-Converter/1

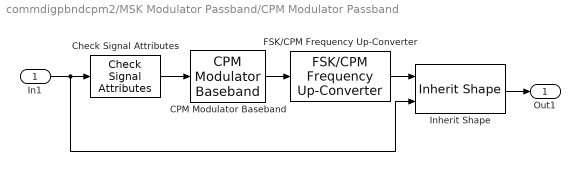
== system commdigpbndcpm2/MSK Modulator Passband/CPM Modulator Passband ==
  In1 : Inport  Port=1  LatchInput=off
  CPM Modulator Baseband : commdigbbndcpm2/CPM Modulator Baseband  Mnum=Mnum  inputType=Integer  mappingType=Binary  modIdx=modIdx  pulseShape=Rectangular  BT=BT  mainLobePulseLength=1  rollOff=rollOff  pulseLength=pulseLength  preHistory=preHistory  phaseOffset=0  samplesPerSymbol=numSamp
  Check Signal Attributes : dspsigattribs/Check Signal Attributes  SigAttribCheckMethod=Matches attributes exactly  Complexity=Ignore  Frame=Frame-based  DimsCheckMethod=Ignore  Dimensions=1-D  DatatypeCheckMethod=Ignore  DatatypeGeneral=Boolean  DtypeFloatSpecific=Any floating-point  DtypeFixedSpecific=Any fixed-point  DtypeIntSpecific=Any integer  SampleMode=Ignore
  FSK/CPM Frequency Up-Converter : commblksprivate/FSK//CPM Frequency Up-Converter  modType=CPM  M=8  freqSep=6  td=td  Fc=Fc  Ph=Ph  Tin=td / numSamp  Tout=OutSamp
  Inherit Shape : commblksprivate/Inherit Shape
  Out1 : Outport  Port=1
  wires:
  Inherit Shape/1 -> Out1/1
  In1/1 -> Inherit Shape/2, Check Signal Attributes/1
  Check Signal Attributes/1 -> CPM Modulator Baseband/1
  CPM Modulator Baseband/1 -> FSK/CPM Frequency Up-Converter/1
  FSK/CPM Frequency Up-Converter/1 -> Inherit Shape/1

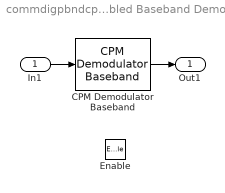
== system commdigpbndcpm2/CPFSK Demodulator Passband/CPM Demodulator Passband/Enabled Baseband Demodulator ==
  In1 : Inport  Port=1  LatchInput=off
  Enable : EnablePort
  CPM Demodulator Baseband : commdigbbndcpm2/CPM Demodulator Baseband  Mnum=Mnum  outputType=Integer  mappingType=Binary  modIdx=modIdx  pulseShape=Rectangular  BT=BT  mainLobePulseLength=1  rollOff=rollOff  pulseLength=pulseLength  preHistory=preHistory  phaseOffset=0  samplesPerSymbol=numSamp  traceBack=traceBack
  Out1 : Outport  Port=1
  wires:
  In1/1 -> CPM Demodulator Baseband/1
  CPM Demodulator Baseband/1 -> Out1/1

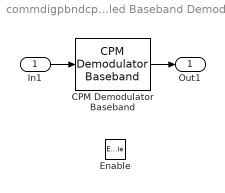
== system commdigpbndcpm2/GMSK Demodulator Passband/CPM Demodulator Passband/Enabled Baseband Demodulator ==
  In1 : Inport  Port=1  LatchInput=off
  Enable : EnablePort
  CPM Demodulator Baseband : commdigbbndcpm2/CPM Demodulator Baseband  Mnum=Mnum  outputType=Integer  mappingType=Binary  modIdx=modIdx  pulseShape=Gaussian  BT=BT  mainLobePulseLength=1  rollOff=rollOff  pulseLength=pulseLength  preHistory=preHistory  phaseOffset=0  samplesPerSymbol=numSamp  traceBack=traceBack
  Out1 : Outport  Port=1
  wires:
  In1/1 -> CPM Demodulator Baseband/1
  CPM Demodulator Baseband/1 -> Out1/1

== system commdigpbndcpm2/MSK Demodulator Passband/CPM Demodulator Passband/Enabled Baseband Demodulator ==
  In1 : Inport  Port=1  LatchInput=off
  Enable : EnablePort
  CPM Demodulator Baseband : commdigbbndcpm2/CPM Demodulator Baseband  Mnum=Mnum  outputType=Integer  mappingType=Binary  modIdx=modIdx  pulseShape=Rectangular  BT=BT  mainLobePulseLength=1  rollOff=rollOff  pulseLength=pulseLength  preHistory=preHistory  phaseOffset=0  samplesPerSymbol=numSamp  traceBack=traceBack
  Out1 : Outport  Port=1
  wires:
  In1/1 -> CPM Demodulator Baseband/1
  CPM Demodulator Baseband/1 -> Out1/1
